simulink model "four_wheeled_inverted_pendulum_lqr"  (R2025a)
settings: Solver=ode45  StartTime=0  StopTime=tEnd  MaxStep=0.005  RelTol=1e-9  AbsTol=1e-9
PreLoadFcn:
  | % Four-Wheeled Inverted Pendulum - parameters (identical to the MATLAB scripts)
  | M = 2.50;  m = 0.50;  l = 0.375;  I = 0.015;  g = 9.81;
  | D = M*(I + m*l^2) - (m*l)^2;
  | A = [0 1 0 0; 0 0 -(g*m^2*l^2)/D 0; 0 0 0 1; 0 0 (M*g*m*l)/D 0];
  | B = [0; (m*l^2 + I)/D; 0; -(m*l)/D];
  | Q = diag([1, 1, 100, 10]);  R = 1;
  | K = lqr(A, B, Q, R);
  | theta0_deg = 5;  X0 = [0; 0; deg2rad(theta0_deg); 0];
  | F_dist_mag = 2.0;  t_dist_start = 2.0;  t_dist_end = 2.2;  tEnd = 5.0;
InitFcn:
  | % Four-Wheeled Inverted Pendulum - parameters (identical to the MATLAB scripts)
  | M = 2.50;  m = 0.50;  l = 0.375;  I = 0.015;  g = 9.81;
  | D = M*(I + m*l^2) - (m*l)^2;
  | A = [0 1 0 0; 0 0 -(g*m^2*l^2)/D 0; 0 0 0 1; 0 0 (M*g*m*l)/D 0];
  | B = [0; (m*l^2 + I)/D; 0; -(m*l)/D];
  | Q = diag([1, 1, 100, 10]);  R = 1;
  | K = lqr(A, B, Q, R);
  | theta0_deg = 5;  X0 = [0; 0; deg2rad(theta0_deg); 0];
  | F_dist_mag = 2.0;  t_dist_start = 2.0;  t_dist_end = 2.2;  tEnd = 5.0;
settings Model: Creator=Naresh Tuppathi  LastModifiedBy=Naresh Tuppathi

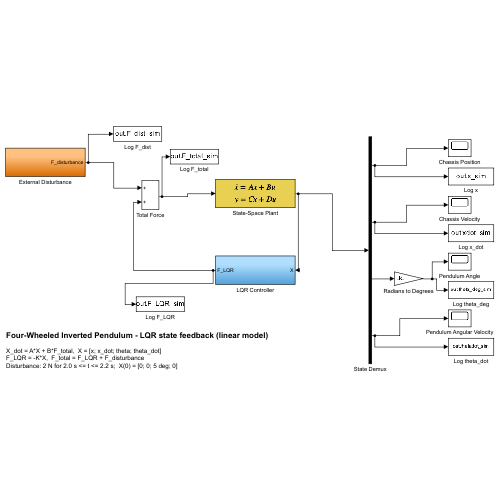
[thumbnail: Simulink's stored preview of the top-level diagram]
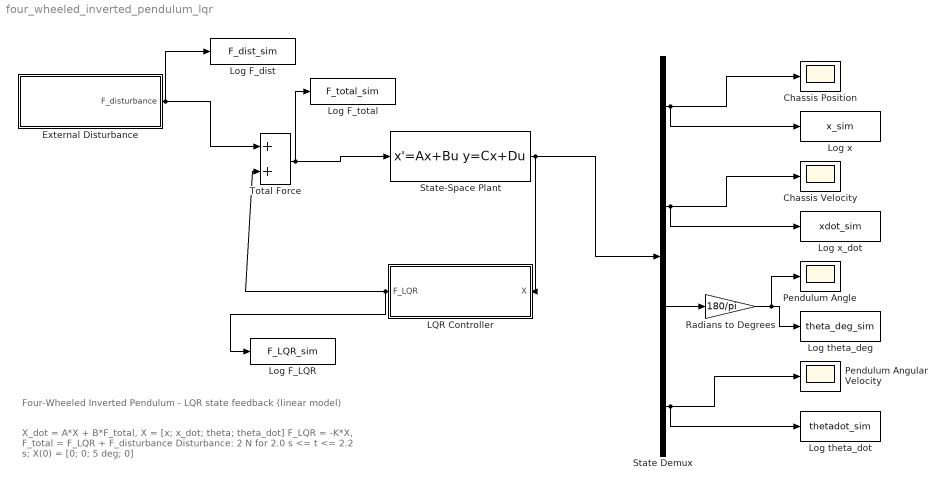
== system four_wheeled_inverted_pendulum_lqr ==
  note: Four-Wheeled Inverted Pendulum - LQR state feedback (linear model)
  note: X_dot = A*X + B*F_total,  X = [x; x_dot; theta; theta_dot]
      | F_LQR = -K*X,  F_total = F_LQR + F_disturbance
      | Disturbance: 2 N for 2.0 s <= t <= 2.2 s;  X(0) = [0; 0; 5 deg; 0]
  Chassis Position : Scope
      settings: Title=Chassis Position x [m]  YLabel=x [m]
  Chassis Velocity : Scope
      settings: Title=Chassis Velocity x_dot [m/s]  YLabel=x_dot [m/s]
  External Disturbance : Subsystem
  LQR Controller : Subsystem
  Log F_LQR : ToWorkspace  VariableName=F_LQR_sim  SaveFormat=Timeseries  SampleTime=-1
  Log F_dist : ToWorkspace  VariableName=F_dist_sim  SaveFormat=Timeseries  SampleTime=-1
  Log F_total : ToWorkspace  VariableName=F_total_sim  SaveFormat=Timeseries  SampleTime=-1
  Log theta_deg : ToWorkspace  VariableName=theta_deg_sim  SaveFormat=Timeseries  SampleTime=-1
  Log theta_dot : ToWorkspace  VariableName=thetadot_sim  SaveFormat=Timeseries  SampleTime=-1
  Log x : ToWorkspace  VariableName=x_sim  SaveFormat=Timeseries  SampleTime=-1
  Log x_dot : ToWorkspace  VariableName=xdot_sim  SaveFormat=Timeseries  SampleTime=-1
  Pendulum Angle : Scope
      settings: Title=Pendulum Angle theta [deg]  YLabel=theta [deg]
  Pendulum Angular Velocity : Scope
      settings: Title=Pendulum Angular Velocity theta_dot [rad/s]  YLabel=theta_dot [rad/s]
  Radians to Degrees : Gain  Gain=180/pi
  State Demux : Demux
  State-Space Plant : StateSpace  A=A  B=B  C=eye(4)  D=zeros(4,1)  InitialCondition=X0
  Total Force : Sum
  wires:
  External Disturbance/1(F_disturbance) -> Total Force/1, Log F_dist/1
  LQR Controller/1(F_LQR) -> Total Force/2, Log F_LQR/1
  Total Force/1 -> State-Space Plant/1, Log F_total/1
  State-Space Plant/1 -> State Demux/1, LQR Controller/1(X)
  State Demux/1 -> Chassis Position/1, Log x/1
  State Demux/2 -> Chassis Velocity/1, Log x_dot/1
  State Demux/3 -> Radians to Degrees/1
  Radians to Degrees/1 -> Pendulum Angle/1, Log theta_deg/1
  State Demux/4 -> Pendulum Angular Velocity/1, Log theta_dot/1

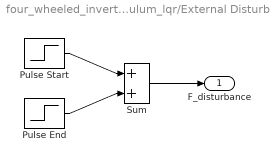
== system four_wheeled_inverted_pendulum_lqr/External Disturbance ==
  Pulse End : Step  Time=t_dist_end  After=-F_dist_mag  SampleTime=0
  Pulse Start : Step  Time=t_dist_start  After=F_dist_mag  SampleTime=0
  Sum : Sum
  F_disturbance : Outport
  wires:
  Pulse Start/1 -> Sum/1
  Pulse End/1 -> Sum/2
  Sum/1 -> F_disturbance/1

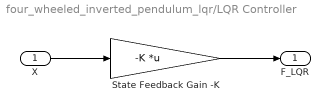
== system four_wheeled_inverted_pendulum_lqr/LQR Controller ==
  X : Inport
  State Feedback Gain -K : Gain  Gain=-K  Multiplication=Matrix(K*u)
  F_LQR : Outport
  wires:
  X/1 -> State Feedback Gain -K/1
  State Feedback Gain -K/1 -> F_LQR/1
